simulink model "QuaterCarModel"  (R2022a)
settings: Solver=VariableStepAuto  StartTime=0.0  StopTime=10.0  RelTol=1e-3
PreLoadFcn:
  | load('variables');
  | 
  | Yr=1;
values from neighbouring files (symbols this model uses):
  Cs = 2500    [variables.mat]
  Ks = 25000    [variables.mat]
  Kt = 200000    [variables.mat]
  Ms = 400    [variables.mat]
  Mus = 30    [variables.mat]
settings Model: Creator=seong  LastModifiedBy=user
settings SolverCC: AlgebraicLoopSolver=TrustRegion
settings DataIOCC: ExternalInput=[Time,RoadProfile]  SaveFormat=Array  ReturnWorkspaceOutputs=off  TimeSaveName=Time1  OutputSaveName=Ys, Yus
settings DebuggingCC: UnconnectedInputMsg=warning  UnconnectedOutputMsg=warning  UnconnectedLineMsg=warning  SFMachineParentedDataDiag=warning
settings SFSimCC: CustomCodeUndefinedFunction=UseInterfaceOnly
settings RTWCC: DLArmComputeVersion=19.05

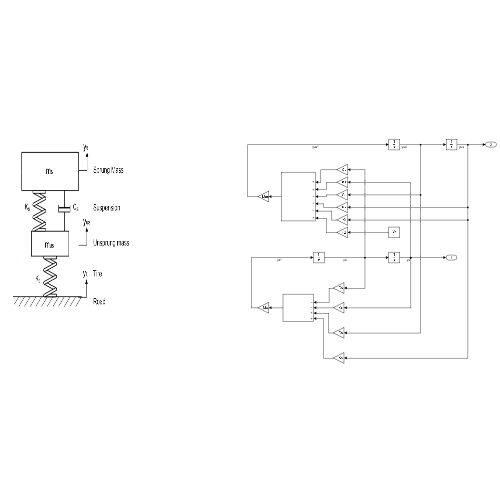
[thumbnail: Simulink's stored preview of the top-level diagram]
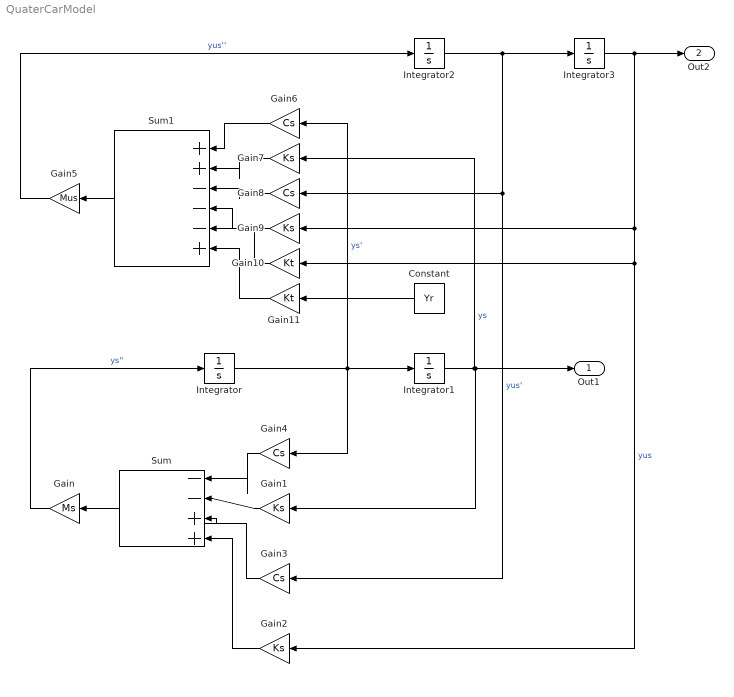
== system QuaterCarModel ==
  Constant : Constant  Value=Yr
  Gain : Gain  Gain=Ms
  Gain{1..2,7,9} (4 alike) : Gain  Gain=Ks
  Gain10 : Gain  Gain=Kt
  Gain11 : Gain  Gain=Kt
  Gain{3..4,6,8} (4 alike) : Gain  Gain=Cs
  Gain5 : Gain  Gain=Mus
  Integrator{,1..3} (4 alike) : Integrator
  Sum : Sum  Inputs=|--++
  Sum1 : Sum  Inputs=|++---+
  Out1 : Outport
  Out2 : Outport  Port=2
  wires:
  Constant/1 -> Gain11/1
  Gain1/1 -> Sum/2
  Sum/1 -> Gain/1
  Gain5/1 -> Integrator2/1  "yus''"
  Gain8/1 -> Sum1/3
  Integrator/1 -> Gain6/1, Gain4/1, Integrator1/1  "ys'"
  Gain10/1 -> Sum1/5
  Gain4/1 -> Sum/1
  Sum1/1 -> Gain5/1
  Integrator3/1 -> Gain9/1, Gain2/1, Gain10/1, Out2/1  "yus"
  Gain6/1 -> Sum1/1
  Gain9/1 -> Sum1/4
  Gain11/1 -> Sum1/6
  Integrator2/1 -> Gain3/1, Gain8/1, Integrator3/1  "yus'"
  Gain3/1 -> Sum/3
  Gain7/1 -> Sum1/2
  Integrator1/1 -> Out1/1, Gain1/1, Gain7/1  "ys"
  Gain/1 -> Integrator/1  "ys''"
  Gain2/1 -> Sum/4
